simulink model "hybrid_controller_handmade_v1"  (R2024b)
settings: Solver=VariableStepAuto  StartTime=0.0  StopTime=45  RelTol=1e-3
values from neighbouring files (symbols this model uses):
  Aobs = A_aug - L*C_aug    [init_eso_ros.m]
  Bobs = [B_aug-L, L]    [init_eso_ros.m]
  Cobs = eye(nx+1)    [init_eso_ros.m]
  Dobs = zeros(nx+1,2)    [init_eso_ros.m]
  nx = size(Ad,1)    [init_eso_ros.m]
  Ts = 0.05    [init_eso_ros.m]
  z0 = zeros(nx+1,1)    [init_eso_ros.m]
libraries: simulink x3, ros2lib x3, mpclib x2, dspstat3 x1, SignalEditorBlockLib x1
settings Model: Creator=kimtaehyeong  LastModifiedBy=samsung

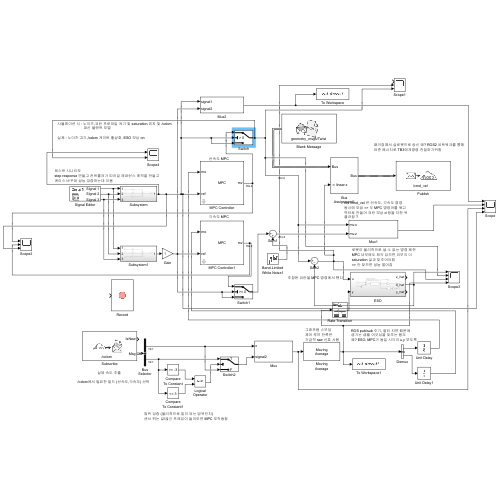
[thumbnail: Simulink's stored preview of the top-level diagram]
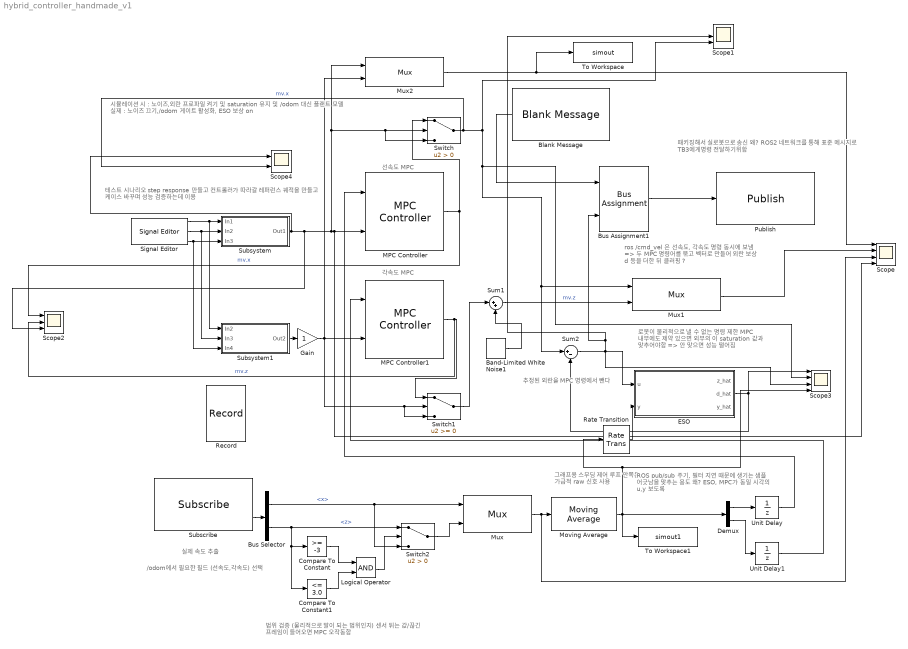
== system hybrid_controller_handmade_v1 ==
  note: 그래프용 스무딩
      | 제어 루프 안쪽은
      | 가급적 raw 신호 사용
  note: 패키징해서 실로봇으로 송신 왜? ROS2 네트워크를 통해
      | 표준 메시지로 TB3에게명령 전달하기위함
  note: ros /cmd_vel 은 선속도, 각속도 명령 동시에 보냄 => 두 MPC 명령어를 묶고
      | 벡터로 만들어 외란 보상 d 등을 더한 뒤
      | 클러핑 ?
  note: 각속도 MPC
  note: 선속도 MPC
  note: 테스트 시나리오
      | step response 만들고 컨트롤러가 따라갈 레퍼런스 궤적을 만들고
      | 케이스 바꾸며 성능 검증하는데 이용
  note: 시뮬레이션 시 : 노이즈,외란 프로파일 켜기 및 saturation 유지 및 /odom
      |                           대신 플랜트 모델
      |
      | 실제 : 노이즈 끄기,/odom 게이트 활성화, ESO 보상 on
  note: 실제 속도 추출
  note: /odom에서 필요한 필드 (선속도,각속도) 선택
  note: 범위 검증 (물리적으로 말이 되는 범위인지)
      | 센서 튀는 값/끊긴 프레임이 들어오면 MPC 오작동함
  note: ROS pub/sub 주기, 필터 지연 때문에
      | 생기는 샘플 어긋남을 맞추는 용도
      | 왜? ESO, MPC가 동일 시각의 u,y 보도록
  note: 추정된 외란을 MPC 명령에서 뺀다
  note: 로봇이 물리적으로 낼 수 없는 명령 제한
      | MPC 내부에도 제약 있으면 외부의 이 saturation 값과 맞추어야함
      | => 안 맞으면 성능 떨어짐
  Band-Limited White Noise1 : simulink/Sources/Band-Limited White Noise  Cov=[0.1]  Ts=0.1  seed=[23341]
  Blank Message : ros2lib/Blank Message  messageClass=Message  entityType=geometry_msgs/Twist  messageType=geometry_msgs/Twist  SampleTime=0.05
  Bus Assignment1 : BusAssignment  AssignedSignals=linear.x
  Bus Selector : BusSelector  OutputSignals=pose.pose.position.x,twist.twist.angular.z
  Compare To Constant : simulink/Logic and Bit Operations/Compare To Constant  relop=>=  const=-3  OutDataTypeStr=boolean
  Compare To Constant1 : simulink/Logic and Bit Operations/Compare To Constant  relop=<=  const=3.0  OutDataTypeStr=boolean
  Demux : Demux  Outputs=2
      settings: DisplayOption=none
  ESO : Subsystem
  Gain : Gain
  Logical Operator : Logic  AllPortsSameDT=off  OutDataTypeStr=boolean
  MPC Controller : mpclib/MPC Controller  SCDEnableBlockLinearizationSpecification=on  mpcobj=mpc_linear  is_multiple=0  enable_value=0  return_u0=off  updateMPCinCallerWorkspace=on  md_inport=off  mv_inport=off  uref_inport=off  return_cost=off  return_mvseq=off  return_qpstatus=off  return_xseq=off  return_state=off  return_ovseq=off  state_inport=off  umin_inport=off  umax_inport=off  ymin_inport=off  ymax_inport=off  cc_inport=off  ywt_inport=off  uwt_inport=off  duwt_inport=off  rhoeps_inport=off  pm_inport=off  MaximumP=10  HorizonChoice=FixedHorizon  n_ts=0.05  n_p=20  n_mv=1  n_md=0  n_ud=0  n_mo=1  n_uo=0  BlockDataType=double  SampleTimeInherited=off  switch_inport=off
  MPC Controller1 : mpclib/MPC Controller  SCDEnableBlockLinearizationSpecification=on  mpcobj=mpc_angular  is_multiple=0  enable_value=0  return_u0=off  updateMPCinCallerWorkspace=on  md_inport=off  mv_inport=off  uref_inport=off  return_cost=off  return_mvseq=off  return_qpstatus=off  return_xseq=off  return_state=off  return_ovseq=off  state_inport=off  umin_inport=off  umax_inport=off  ymin_inport=off  ymax_inport=off  cc_inport=off  ywt_inport=off  uwt_inport=off  duwt_inport=off  rhoeps_inport=off  pm_inport=off  MaximumP=10  HorizonChoice=FixedHorizon  n_ts=0.05  n_p=10  n_mv=1  n_md=0  n_ud=0  n_mo=1  n_uo=0  BlockDataType=double  SampleTimeInherited=off  switch_inport=off
  Moving Average : dspstat3/Moving Average  Method=Sliding window  ForgettingFactorPort=off  SpecifyWindowLength=on  WindowLength=4  OverlapLength=3  AllowArbitraryInputLength=off  ForgettingFactor=0.9  SimulateUsing=Interpreted execution
  Mux : Mux  Inputs=2
      settings: DisplayOption=signals
  Mux1 : Mux  Inputs=2
      settings: DisplayOption=signals
  Mux2 : Mux  Inputs=2
      settings: DisplayOption=signals
  Publish : ros2lib/Publish  topicSource=Specify your own  topic=/cmd_vel  messageType=geometry_msgs/Twist  QOSHistory=Keep last  QOSDepth=1  QOSReliability=Reliable  QOSDurability=Volatile  QOSDeadline=Inf  QOSLifespan=Inf  QOSLiveliness=Automatic  QOSLeaseDuration=Inf  QOSAvoidROSNamespaceConventions=off
  Rate Transition : RateTransition  OutPortSampleTime=0.05
  Record : Record  FileSettingsInternal="{\"entries\":[{\"content\":{\"excelSettings\":{\"content\":{},\"type\":\"Streamout.ExcelSettings\"}},\"type\":\"Streamout.FileSettingStorage\",\"uuid\":\"\"}],\"packageUris\":[\"http:\\/\\/schema.mathworks.com\\/mf0\\/streamout_blocks\\/R2020a\"],\"version\":\"1.0\"}"  SignalsInternal="{\"entries\":[{\"content\":{\"signals\":[{\"content\":{\"blockPath\":[],\"dimensions\":[1],\"domain\":\"\",\"lineColor\":\"#edb120\",\"lineWidth\":2,\"plots\":[ 1 ],\"port\":1,\"sid\":[\"\"],\"signalID\":1},\"type\":\"RecordBlkView.Signal\",\"uuid\":\"\"}]},\"type\":\"RecordBlkView.InputSignals\",\"uuid\":\"\"}],\"packageUris\":[\"http:\\/\\/schema.mathworks.com\\/mf0\\/streamout_blocks\\/R2020a\"],\"version\":\"1.0\"}"  VisualizationBindings="{\"sparklinesplugin\":{\"info\":[{\"bindingParametersList\":[],\"subplotID\":1}]}}"
  Scope : Scope  NumInputPorts=4
  Scope1 : Scope  NumInputPorts=3
  Scope2 : Scope  NumInputPorts=3
  Scope3 : Scope  NumInputPorts=4
  Scope4 : Scope  NumInputPorts=2
  Signal Editor : SignalEditorBlockLib/Signal Editor  FileName=D:\Users\rladm\OneDrive\문서\MATLAB\FOMPC_PID\mpc\signal_handmade.mat  ActiveScenario=Group1  ActiveSignal=Signal 1  IsBus=off  OutputBusObjectStr=Bus: BusObject  SampleTime=0.05  Interpolate=off  ZeroCross=off  OutputAfterFinalValue=Setting to zero  Unit=m/s  PreserveSignalName=on  ApplySigPropsToAllScenarios=on  ApplySigPropsToAllSignals=off
  Subscribe : ros2lib/Subscribe  topicSource=Specify your own  topic=/odom  messageType=nav_msgs/Odometry  sampleTime=0.05  QOSHistory=Keep last  QOSDepth=1  QOSReliability=Reliable  QOSDurability=Volatile  QOSDeadline=Inf  QOSLifespan=Inf  QOSLiveliness=Automatic  QOSLeaseDuration=Inf  QOSAvoidROSNamespaceConventions=off
  Subsystem : Subsystem
  Subsystem1 : Subsystem
  Sum1 : Sum  Inputs=|++
  Sum2 : Sum  Inputs=|+-
  Switch : Switch  Criteria=u2 > Threshold  SaturateOnIntegerOverflow=off  InputSameDT=off
  Switch1 : Switch  SaturateOnIntegerOverflow=off  InputSameDT=off
  Switch2 : Switch  Criteria=u2 > Threshold  OutDataTypeStr=double  SaturateOnIntegerOverflow=off
  To Workspace : ToWorkspace  VariableName=simout  SaveFormat=Timeseries  SampleTime=-1
  To Workspace1 : ToWorkspace  VariableName=simout1  SaveFormat=Timeseries  SampleTime=-1
  Unit Delay : UnitDelay  SampleTime=-1  HasFrameUpgradeWarning=on
  Unit Delay1 : UnitDelay  SampleTime=-1  HasFrameUpgradeWarning=on
  wires:
  Signal Editor/1 -> Subsystem1/1(In2), Subsystem/1(In1)
  Signal Editor/2 -> Subsystem1/2(In3), Subsystem/2(In2)
  Signal Editor/3 -> Subsystem1/3(In4), Subsystem/3(In3)
  Subsystem1/1(Out2) -> Gain/1
  Gain/1 -> Switch1/3, Switch1/2, Mux2/2, MPC Controller1/2
  Subsystem/1(Out1) -> Scope4/1, Scope/4, MPC Controller/2, Switch/3, Switch/2, Mux2/1, Scope2/3
  MPC Controller/1 -> Switch/1, Scope2/1  "mv.x"
  MPC Controller1/1 -> Scope2/2, Switch1/1  "mv.z"
  Switch1/1 -> Sum1/1
  Band-Limited White Noise1/1 -> Sum1/2
  Switch/1 -> Scope4/2, Sum2/1, Mux1/1, Scope3/2, Scope1/3  "mv.x"
  Subscribe/2 -> Bus Selector/1
  Compare To Constant/1 -> Logical Operator/1
  Compare To Constant1/1 -> Logical Operator/2
  Logical Operator/1 -> Switch2/2
  Bus Assignment1/1 -> Publish/1
  Blank Message/1 -> Bus Assignment1/1
  Sum1/1 -> Mux1/2  "mv.z"
  Switch2/1 -> Mux/2
  Bus Selector/2 -> Compare To Constant/1, Compare To Constant1/1, Switch2/1  "<z>"
  Bus Selector/1 -> Mux/1, Switch2/3  "<x>"
  Mux2/1 -> Scope/1, To Workspace/1
  Mux1/1 -> Scope/2
  Demux/1 -> Unit Delay/1
  Demux/2 -> Unit Delay1/1
  Mux/1 -> Moving Average/1, Scope/3
  Moving Average/1 -> To Workspace1/1, Scope3/4, Rate Transition/1, Demux/1
  Unit Delay/1 -> MPC Controller/1
  Unit Delay1/1 -> MPC Controller1/1
  ESO/2(d_hat) -> Scope3/1, Sum2/2
  Sum2/1 -> Bus Assignment1/2, Scope1/2, Scope3/3, ESO/1(u)
  Rate Transition/1 -> ESO/2(y)

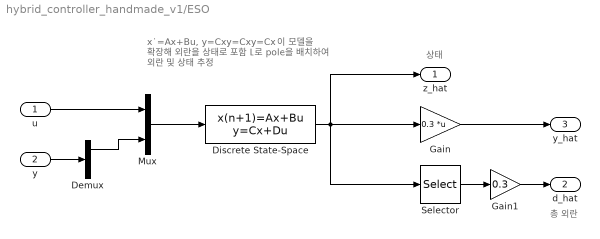
== system hybrid_controller_handmade_v1/ESO ==
  note: 상태
  note: 총 외란
  note: x˙=Ax+Bu, y=Cxy=Cxy=Cx
      | 이 모델을 확장해 외란을 상태로 포함
      | L로 pole을 배치하여 외란 및 상태 추정
  u : Inport
  y : Inport  Port=2
  Demux : Demux  Outputs=2
  Discrete State-Space : DiscreteStateSpace  A=Aobs  B=Bobs  C=Cobs  D=Dobs  InitialCondition=z0  SampleTime=Ts
  Gain : Gain  Gain=0.3  Multiplication=Matrix(K*u)
  Gain1 : Gain  Gain=0.3
  Mux : Mux  Inputs=2
      settings: DisplayOption=signals
  Selector : Selector  IndexOptions=Index vector (dialog)  Indices=nx+1  OutputSizes=1
  z_hat : Outport
  d_hat : Outport  Port=2
  y_hat : Outport  Port=3
  wires:
  u/1 -> Mux/1
  Mux/1 -> Discrete State-Space/1
  Discrete State-Space/1 -> Selector/1, z_hat/1, Gain/1
  Gain/1 -> y_hat/1
  y/1 -> Demux/1
  Demux/1 -> Mux/2
  Selector/1 -> Gain1/1
  Gain1/1 -> d_hat/1

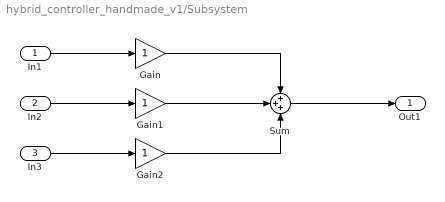
== system hybrid_controller_handmade_v1/Subsystem ==
  In1 : Inport
  In2 : Inport  Port=2
  In3 : Inport  Port=3
  Gain : Gain
  Gain1 : Gain
  Gain2 : Gain
  Sum : Sum  Inputs=+++
  Out1 : Outport
  wires:
  Gain/1 -> Sum/1
  Gain1/1 -> Sum/2
  Gain2/1 -> Sum/3
  In1/1 -> Gain/1
  In2/1 -> Gain1/1
  In3/1 -> Gain2/1
  Sum/1 -> Out1/1

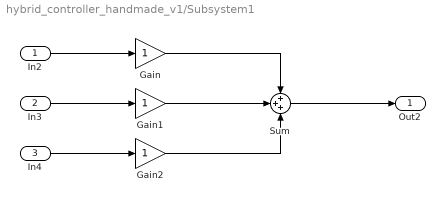
== system hybrid_controller_handmade_v1/Subsystem1 ==
  In2 : Inport
  In3 : Inport  Port=2
  In4 : Inport  Port=3
  Gain : Gain
  Gain1 : Gain
  Gain2 : Gain
  Sum : Sum  Inputs=+++
  Out2 : Outport
  wires:
  In2/1 -> Gain/1
  In4/1 -> Gain2/1
  In3/1 -> Gain1/1
  Gain1/1 -> Sum/2
  Gain2/1 -> Sum/3
  Gain/1 -> Sum/1
  Sum/1 -> Out2/1
